simulink model "gm_hybrid_lht_vnl"  (R2019b)
settings: Solver=FixedStepDiscrete  StartTime=0.0  StopTime=inf  FixedStep=1/120e6  RelTol=1e-3
undefined symbols (not defined in the file or in its folder): bt, height, nTheta, width
libraries: hdlsllib x252, simulink x168, hdlmdlgenlib x11, dspsrcs4 x1
(part 10 of 12)

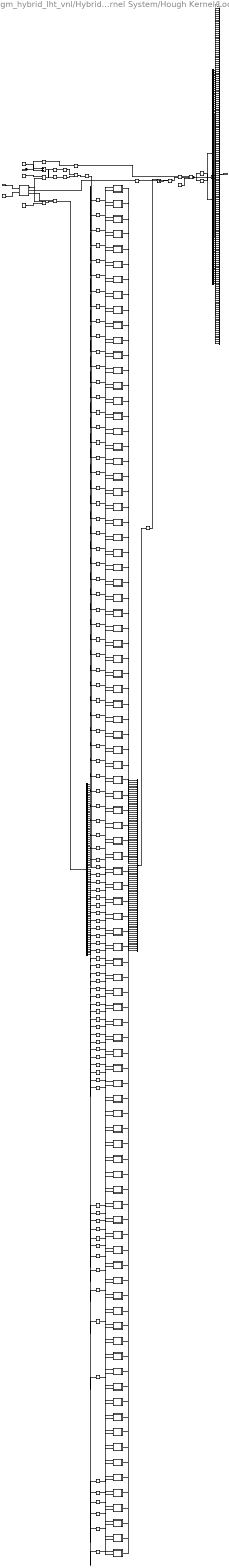
== system gm_hybrid_lht_vnl/Hybrid LHT/Hybrid LHT Kernel/Gradient Kernel System/Hough Kernel/Look Ahead Hough/Look Ahead Hough Symmetric ==
  Y : Inport  OutDataTypeStr=int8  PortDimensions=1  SampleTime=8.33333333333333e-09
  eol : Inport  Port=2  OutDataTypeStr=boolean  PortDimensions=1  SampleTime=8.33333333333333e-09
  AND1 : Logic  AllPortsSameDT=off  OutDataTypeStr=boolean  SampleTime=8.33333333333333e-09
  Add : Sum  AccumDataTypeStr=int8  OutDataTypeStr=int8  SampleTime=8.33333333333333e-09
  Compare To Constant : simulink/Logic and Bit Operations/Compare To Constant  relop===  const=fi(0,1,8,0,'hex','88')  OutDataTypeStr=boolean
  Constant : Constant  Value=90  OutDataTypeStr=uint8  SampleTime=-1
  Constant1 : Constant  OutDataTypeStr=int8  SampleTime=-1
  Delay_Switch : Switch  Criteria=u2 ~= 0  Threshold=double(0)  OutDataTypeStr=int8  SampleTime=8.33333333333333e-09
  HwModeRegister : Delay  DelayLength=double(1)  InitialCondition=0  SampleTime=8.33333333333333e-09
  HwModeRegister1 : Delay  DelayLength=double(1)  InitialCondition=0  SampleTime=8.33333333333333e-09
  MATLAB Function : Subsystem
  Multiport Switch : MultiPortSwitch  DataPortOrder=Zero-based contiguous  Inputs=2  DiagnosticForDefault=None  zeroidx=on  OutDataTypeStr=int8  SampleTime=8.33333333333333e-09
  PipelineRegister : Delay  DelayLength=double(1)  InitialCondition=0  SampleTime=8.33333333333333e-09
  Register Bank_instance1 : Subsystem
  Register Bank_instance10 : Subsystem
  Register Bank_instance11 : Subsystem
  Register Bank_instance12 : Subsystem
  Register Bank_instance13 : Subsystem
  Register Bank_instance14 : Subsystem
  Register Bank_instance15 : Subsystem
  Register Bank_instance16 : Subsystem
  Register Bank_instance17 : Subsystem
  Register Bank_instance18 : Subsystem
  Register Bank_instance19 : Subsystem
  Register Bank_instance2 : Subsystem
  Register Bank_instance20 : Subsystem
  Register Bank_instance21 : Subsystem
  Register Bank_instance22 : Subsystem
  Register Bank_instance23 : Subsystem
  Register Bank_instance24 : Subsystem
  Register Bank_instance25 : Subsystem
  Register Bank_instance26 : Subsystem
  Register Bank_instance27 : Subsystem
  Register Bank_instance28 : Subsystem
  Register Bank_instance29 : Subsystem
  Register Bank_instance3 : Subsystem
  Register Bank_instance30 : Subsystem
  Register Bank_instance31 : Subsystem
  Register Bank_instance32 : Subsystem
  Register Bank_instance33 : Subsystem
  Register Bank_instance34 : Subsystem
  Register Bank_instance35 : Subsystem
  Register Bank_instance36 : Subsystem
  Register Bank_instance37 : Subsystem
  Register Bank_instance38 : Subsystem
  Register Bank_instance39 : Subsystem
  Register Bank_instance4 : Subsystem
  Register Bank_instance40 : Subsystem
  Register Bank_instance41 : Subsystem
  Register Bank_instance42 : Subsystem
  Register Bank_instance43 : Subsystem
  Register Bank_instance44 : Subsystem
  Register Bank_instance45 : Subsystem
  Register Bank_instance46 : Subsystem
  Register Bank_instance47 : Subsystem
  Register Bank_instance48 : Subsystem
  Register Bank_instance49 : Subsystem
  Register Bank_instance5 : Subsystem
  Register Bank_instance50 : Subsystem
  Register Bank_instance51 : Subsystem
  Register Bank_instance52 : Subsystem
  Register Bank_instance53 : Subsystem
  Register Bank_instance54 : Subsystem
  Register Bank_instance55 : Subsystem
  Register Bank_instance56 : Subsystem
  Register Bank_instance57 : Subsystem
  Register Bank_instance58 : Subsystem
  Register Bank_instance59 : Subsystem
  Register Bank_instance6 : Subsystem
  Register Bank_instance60 : Subsystem
  Register Bank_instance61 : Subsystem
  Register Bank_instance62 : Subsystem
  Register Bank_instance63 : Subsystem
  Register Bank_instance64 : Subsystem
  Register Bank_instance65 : Subsystem
  Register Bank_instance66 : Subsystem
  Register Bank_instance67 : Subsystem
  Register Bank_instance68 : Subsystem
  Register Bank_instance69 : Subsystem
  Register Bank_instance7 : Subsystem
  Register Bank_instance70 : Subsystem
  Register Bank_instance71 : Subsystem
  Register Bank_instance72 : Subsystem
  Register Bank_instance73 : Subsystem
  Register Bank_instance74 : Subsystem
  Register Bank_instance75 : Subsystem
  Register Bank_instance76 : Subsystem
  Register Bank_instance77 : Subsystem
  Register Bank_instance78 : Subsystem
  Register Bank_instance79 : Subsystem
  Register Bank_instance8 : Subsystem
  Register Bank_instance80 : Subsystem
  Register Bank_instance81 : Subsystem
  Register Bank_instance82 : Subsystem
  Register Bank_instance83 : Subsystem
  Register Bank_instance84 : Subsystem
  Register Bank_instance85 : Subsystem
  Register Bank_instance86 : Subsystem
  Register Bank_instance87 : Subsystem
  Register Bank_instance88 : Subsystem
  Register Bank_instance89 : Subsystem
  Register Bank_instance9 : Subsystem
  Register Bank_instance90 : Subsystem
  Register Bank_instance91 : Subsystem
  Relational Operator : RelationalOperator  Operator===  OutDataTypeStr=boolean  SampleTime=8.33333333333333e-09  RndMeth=Nearest
  Selector : Selector  NumberOfDimensions=2  IndexMode=Zero-based  SampleTime=8.33333333333333e-09  IndexOptions=Index vector (dialog),Index vector (dialog)  Indices=double(0),double(90)  OutputSizes=double(1),double(1)
  Selector1 : Selector  NumberOfDimensions=2  IndexMode=Zero-based  SampleTime=8.33333333333333e-09  IndexOptions=Index vector (dialog),Index vector (port)  Indices=double(0),double(1)  OutputSizes=double(1),double(1)
  Selector2 : Selector  NumberOfDimensions=2  IndexMode=Zero-based  SampleTime=8.33333333333333e-09  IndexOptions=Index vector (dialog),Index vector (dialog)  Indices=double(0),double([0 1 2 3 4 5 6 7 8 9 10 11 12 13 14 15 16 17 18 19 20 21 22 23 24 25 26 27 28 29 30 31 32 33 34 35 36 37 38 39 40 41 42 43 44 45 46 47 48 49 50 51 52 53 54 55 56 57 58 59 60 61 62 63 64 65 66 67 68 69 70 71 72 73 74 75 76 77 78 79 80 81 82 83 84 85 86 87 88 89])  OutputSizes=double(1),double(1)
  Selector3 : Selector  NumberOfDimensions=2  IndexMode=Zero-based  SampleTime=8.33333333333333e-09  IndexOptions=Index vector (dialog),Index vector (dialog)  Indices=double(0),double([89 88 87 86 85 84 83 82 81 80 79 78 77 76 75 74 73 72 71 70 69 68 67 66 65 64 63 62 61 60 59 58 57 56 55 54 53 52 51 50 49 48 47 46 45 44 43 42 41 40 39 38 37 36 35 34 33 32 31 30 29 28 27 26 25 24 23 22 21 20 19 18 17 16 15 14 13 12 11 10 9 8 7 6 5 4 3 2 1])  OutputSizes=double(1),double(1)
  SineROM : Constant  Value=[0 0.0174560546875 0.034912109375 0.05230712890625 0.06976318359375 0.087158203125 0.10455322265625 0.12188720703125 0.13916015625 0.15643310546875 0.17364501953125 0.1907958984375 0.2078857421875 0.2249755859375 0.241943359375 0.2587890625 0.275634765625 0.2923583984375 0.30902099609375 0.3255615234375 0.342041015625 0.3583984375 0.3746337890625 0.3907470703125 0.40673828125 0.422607421875 0.4383544921875 0.4539794921875 0.469482421875 0.48480224609375 0.5 0.5150146484375 0.5299072265625 0.54461669921875 0.5592041015625 0.57354736328125 0.5877685546875 0.601806640625 0.61566162109375 0.62933349609375 0.64276123046875 0.65606689453125 0.66912841796875 0.6820068359375 0.69464111328125 0.70709228515625 0.7193603515625 0.7313232421875 0.7431640625 0.75469970703125 0.76605224609375 0.77716064453125 0.78802490234375 0.79864501953125 0.80902099609375 0.81915283203125 0.82904052734375 0.83868408203125 0.8480224609375 0.857177734375 0.86602783203125 0.8746337890625 0.8829345703125 0.8909912109375 0.8988037109375 0.90631103515625 0.91357421875 0.9205322265625 0.92718505859375 0.93359375 0.939697265625 0.94549560546875 0.9510498046875 0.956298828125 0.96124267578125 0.9659423828125 0.97027587890625 0.974365234375 0.9781494140625 0.98162841796875 0.98480224609375 0.9876708984375 0.99029541015625 0.9925537109375 0.9945068359375 0.9962158203125 0.99755859375 0.9986572265625 0.9993896484375 0.9998779296875 1]  VectorParams1D=off  OutDataTypeStr=fixdt(1, 16, 14)  SampleTime=-1
  Unit Delay Enabled Synchronous_lowered : Delay  DelayLength=double(1)  InitialCondition=0  SampleTime=8.33333333333333e-09
  Unit Delay Enabled Synchronous_out1 : hdlmdlgenlib/Buffer
      settings: SourceProductName=Simulink  SourceProductBaseCode=SL
  concatenate : Concatenate  NumInputs=180  Mode=Multidimensional array  ConcatenateDimension=2
  delayMatch{,1..92} (93 alike) : Delay  DelayLength=double(2)  InitialCondition=0  SampleTime=8.33333333333333e-09
  multiply : Product  Inputs=**  OutDataTypeStr=fixdt(1, 24, 14)  SampleTime=8.33333333333333e-09
  multiply_in0_buff : hdlmdlgenlib/Buffer
      settings: SourceProductName=Simulink  SourceProductBaseCode=SL
  multiply_in1_buff : hdlmdlgenlib/Buffer
      settings: SourceProductName=Simulink  SourceProductBaseCode=SL
  multiply_out_dtc : DataTypeConversion  OutDataTypeStr=int8  RndMeth=Round  SampleTime=8.33333333333333e-09
  row_0 : Constant  Value=[0 -2 -4 -6 -8 -10 -13 -15 -17 -19 -21 -23 -25 -27 -29 -31 -33 -35 -37 -39 -41 -43 -45 -47 -49 -51 -53 -54 -56 -58 -60 -62 -64 -65 -67 -69 -71 -72 -74 -76 -77 -79 -80 -82 -83 -85 -86 -88 -89 -91 -92 -93 -95 -96 -97 -98 -99 -101 -102 -103 -104 -105 -106 -107 -108 -109 -110 -110 -111 -112 -113 -113 -114 -115 -115 -116 -116 -117 -117 -118 -118 -119 -119 -119 -119 -120 -120 -120 -120 -120 -120]  VectorParams1D=off  OutDataTypeStr=int8  SampleTime=-1
  t : Demux  Outputs=89
  t1 : Demux  Outputs=90
  t2 : Concatenate  NumInputs=91
  t3 : Reshape  OutputDimensionality=Row vector (2-D)
  t4 : Demux  Outputs=91
  theta_index : Constant  Value=[0 1 2 3 4 5 6 7 8 9 10 11 12 13 14 15 16 17 18 19 20 21 22 23 24 25 26 27 28 29 30 31 32 33 34 35 36 37 38 39 40 41 42 43 44 45 46 47 48 49 50 51 52 53 54 55 56 57 58 59 60 61 62 63 64 65 66 67 68 69 70 71 72 73 74 75 76 77 78 79 80 81 82 83 84 85 86 87 88 89 90]  VectorParams1D=off  OutDataTypeStr=uint8  SampleTime=-1
  ysin : Outport  VectorParamsAs1DForOutWhenUnconnected=off
  wires:
  multiply_in1_buff/1 -> HwModeRegister1/1
  multiply_in0_buff/1 -> HwModeRegister/1
  HwModeRegister1/1 -> multiply/2
  HwModeRegister/1 -> multiply/1
  multiply/1 -> PipelineRegister/1
  t2/1 -> t3/1
  t1/90 -> concatenate/90
  t1/89 -> concatenate/89
  t1/88 -> concatenate/88
  t1/87 -> concatenate/87
  t1/86 -> concatenate/86
  t1/85 -> concatenate/85
  t1/84 -> concatenate/84
  t1/83 -> concatenate/83
  t1/82 -> concatenate/82
  t1/81 -> concatenate/81
  t1/80 -> concatenate/80
  t1/79 -> concatenate/79
  t1/78 -> concatenate/78
  t1/77 -> concatenate/77
  t1/76 -> concatenate/76
  t1/75 -> concatenate/75
  t1/74 -> concatenate/74
  t1/73 -> concatenate/73
  t1/72 -> concatenate/72
  t1/71 -> concatenate/71
  t1/70 -> concatenate/70
  t1/69 -> concatenate/69
  t1/68 -> concatenate/68
  t1/67 -> concatenate/67
  t1/66 -> concatenate/66
  t1/65 -> concatenate/65
  t1/64 -> concatenate/64
  t1/63 -> concatenate/63
  t1/62 -> concatenate/62
  t1/61 -> concatenate/61
  t1/60 -> concatenate/60
  t1/59 -> concatenate/59
  t1/58 -> concatenate/58
  t1/57 -> concatenate/57
  t1/56 -> concatenate/56
  t1/55 -> concatenate/55
  t1/54 -> concatenate/54
  t1/53 -> concatenate/53
  t1/52 -> concatenate/52
  t1/51 -> concatenate/51
  t1/50 -> concatenate/50
  t1/49 -> concatenate/49
  t1/48 -> concatenate/48
  t1/47 -> concatenate/47
  t1/46 -> concatenate/46
  t1/45 -> concatenate/45
  t1/44 -> concatenate/44
  t1/43 -> concatenate/43
  t1/42 -> concatenate/42
  t1/41 -> concatenate/41
  t1/40 -> concatenate/40
  t1/39 -> concatenate/39
  t1/38 -> concatenate/38
  t1/37 -> concatenate/37
  t1/36 -> concatenate/36
  t1/35 -> concatenate/35
  t1/34 -> concatenate/34
  t1/33 -> concatenate/33
  t1/32 -> concatenate/32
  t1/31 -> concatenate/31
  t1/30 -> concatenate/30
  t1/29 -> concatenate/29
  t1/28 -> concatenate/28
  t1/27 -> concatenate/27
  t1/26 -> concatenate/26
  t1/25 -> concatenate/25
  t1/24 -> concatenate/24
  t1/23 -> concatenate/23
  t1/22 -> concatenate/22
  t1/21 -> concatenate/21
  t1/20 -> concatenate/20
  t1/19 -> concatenate/19
  t1/18 -> concatenate/18
  t1/17 -> concatenate/17
  t1/16 -> concatenate/16
  t1/15 -> concatenate/15
  t1/14 -> concatenate/14
  t1/13 -> concatenate/13
  t1/12 -> concatenate/12
  t1/11 -> concatenate/11
  t1/10 -> concatenate/10
  t1/9 -> concatenate/9
  t1/8 -> concatenate/8
  t1/7 -> concatenate/7
  t1/6 -> concatenate/6
  t1/5 -> concatenate/5
  t1/4 -> concatenate/4
  t1/3 -> concatenate/3
  t1/2 -> concatenate/2
  t1/1 -> concatenate/1
  t/89 -> concatenate/180
  t/88 -> concatenate/179
  t/87 -> concatenate/178
  t/86 -> concatenate/177
  t/85 -> concatenate/176
  t/84 -> concatenate/175
  t/83 -> concatenate/174
  t/82 -> concatenate/173
  t/81 -> concatenate/172
  t/80 -> concatenate/171
  t/79 -> concatenate/170
  t/78 -> concatenate/169
  t/77 -> concatenate/168
  t/76 -> concatenate/167
  t/75 -> concatenate/166
  t/74 -> concatenate/165
  t/73 -> concatenate/164
  t/72 -> concatenate/163
  t/71 -> concatenate/162
  t/70 -> concatenate/161
  t/69 -> concatenate/160
  t/68 -> concatenate/159
  t/67 -> concatenate/158
  t/66 -> concatenate/157
  t/65 -> concatenate/156
  t/64 -> concatenate/155
  t/63 -> concatenate/154
  t/62 -> concatenate/153
  t/61 -> concatenate/152
  t/60 -> concatenate/151
  t/59 -> concatenate/150
  t/58 -> concatenate/149
  t/57 -> concatenate/148
  t/56 -> concatenate/147
  t/55 -> concatenate/146
  t/54 -> concatenate/145
  t/53 -> concatenate/144
  t/52 -> concatenate/143
  t/51 -> concatenate/142
  t/50 -> concatenate/141
  t/49 -> concatenate/140
  t/48 -> concatenate/139
  t/47 -> concatenate/138
  t/46 -> concatenate/137
  t/45 -> concatenate/136
  t/44 -> concatenate/135
  t/43 -> concatenate/134
  t/42 -> concatenate/133
  t/41 -> concatenate/132
  t/40 -> concatenate/131
  t/39 -> concatenate/130
  t/38 -> concatenate/129
  t/37 -> concatenate/128
  t/36 -> concatenate/127
  t/35 -> concatenate/126
  t/34 -> concatenate/125
  t/33 -> concatenate/124
  t/32 -> concatenate/123
  t/31 -> concatenate/122
  t/30 -> concatenate/121
  t/29 -> concatenate/120
  t/28 -> concatenate/119
  t/27 -> concatenate/118
  t/26 -> concatenate/117
  t/25 -> concatenate/116
  t/24 -> concatenate/115
  t/23 -> concatenate/114
  t/22 -> concatenate/113
  t/21 -> concatenate/112
  t/20 -> concatenate/111
  t/19 -> concatenate/110
  t/18 -> concatenate/109
  t/17 -> concatenate/108
  t/16 -> concatenate/107
  t/15 -> concatenate/106
  t/14 -> concatenate/105
  t/13 -> concatenate/104
  t/12 -> concatenate/103
  t/11 -> concatenate/102
  t/10 -> concatenate/101
  t/9 -> concatenate/100
  t/8 -> concatenate/99
  t/7 -> concatenate/98
  t/6 -> concatenate/97
  t/5 -> concatenate/96
  t/4 -> concatenate/95
  t/3 -> concatenate/94
  t/2 -> concatenate/93
  t/1 -> concatenate/92
  Register Bank_instance1/1(Data Out) -> t2/1
  Register Bank_instance2/1(Data Out) -> t2/2
  multiply_out_dtc/1 -> Register Bank_instance1/1(Data In), Register Bank_instance2/1(Data In), Register Bank_instance3/1(Data In), Register Bank_instance4/1(Data In), Register Bank_instance5/1(Data In), Register Bank_instance6/1(Data In), Register Bank_instance7/1(Data In), Register Bank_instance8/1(Data In), Register Bank_instance9/1(Data In), Register Bank_instance10/1(Data In), Register Bank_instance11/1(Data In), Register Bank_instance12/1(Data In), Register Bank_instance13/1(Data In), Register Bank_instance14/1(Data In), Register Bank_instance15/1(Data In), Register Bank_instance16/1(Data In), Register Bank_instance17/1(Data In), Register Bank_instance18/1(Data In), Register Bank_instance19/1(Data In), Register Bank_instance20/1(Data In), Register Bank_instance21/1(Data In), Register Bank_instance22/1(Data In), Register Bank_instance23/1(Data In), Register Bank_instance24/1(Data In), Register Bank_instance25/1(Data In), Register Bank_instance26/1(Data In), Register Bank_instance27/1(Data In), Register Bank_instance28/1(Data In), Register Bank_instance29/1(Data In), Register Bank_instance30/1(Data In), Register Bank_instance31/1(Data In), Register Bank_instance32/1(Data In), Register Bank_instance33/1(Data In), Register Bank_instance34/1(Data In), Register Bank_instance35/1(Data In), Register Bank_instance36/1(Data In), Register Bank_instance37/1(Data In), Register Bank_instance38/1(Data In), Register Bank_instance39/1(Data In), Register Bank_instance40/1(Data In), Register Bank_instance41/1(Data In), Register Bank_instance42/1(Data In), Register Bank_instance43/1(Data In), Register Bank_instance44/1(Data In), Register Bank_instance45/1(Data In), Register Bank_instance46/1(Data In), Register Bank_instance47/1(Data In), Register Bank_instance48/1(Data In), Register Bank_instance49/1(Data In), Register Bank_instance50/1(Data In), Register Bank_instance51/1(Data In), Register Bank_instance52/1(Data In), Register Bank_instance53/1(Data In), Register Bank_instance54/1(Data In), Register Bank_instance55/1(Data In), Register Bank_instance56/1(Data In), Register Bank_instance57/1(Data In), Register Bank_instance58/1(Data In), Register Bank_instance59/1(Data In), Register Bank_instance60/1(Data In), Register Bank_instance61/1(Data In), Register Bank_instance62/1(Data In), Register Bank_instance63/1(Data In), Register Bank_instance64/1(Data In), Register Bank_instance65/1(Data In), Register Bank_instance66/1(Data In), Register Bank_instance67/1(Data In), Register Bank_instance68/1(Data In), Register Bank_instance69/1(Data In), Register Bank_instance70/1(Data In), Register Bank_instance71/1(Data In), Register Bank_instance72/1(Data In), Register Bank_instance73/1(Data In), Register Bank_instance74/1(Data In), Register Bank_instance75/1(Data In), Register Bank_instance76/1(Data In), Register Bank_instance77/1(Data In), Register Bank_instance78/1(Data In), Register Bank_instance79/1(Data In), Register Bank_instance80/1(Data In), Register Bank_instance81/1(Data In), Register Bank_instance82/1(Data In), Register Bank_instance83/1(Data In), Register Bank_instance84/1(Data In), Register Bank_instance85/1(Data In), Register Bank_instance86/1(Data In), Register Bank_instance87/1(Data In), Register Bank_instance88/1(Data In), Register Bank_instance89/1(Data In), Register Bank_instance90/1(Data In), Register Bank_instance91/1(Data In)
  PipelineRegister/1 -> multiply_out_dtc/1
  Add/1 -> multiply_in1_buff/1
  Selector1/1 -> multiply_in0_buff/1
  Register Bank_instance91/1(Data Out) -> t2/91
  delayMatch92/1 -> Register Bank_instance91/2(Write Enable)
  t4/91 -> delayMatch92/1
  t4/90 -> delayMatch91/1
  t4/89 -> delayMatch90/1
  t4/88 -> delayMatch89/1
  t4/87 -> delayMatch88/1
  t4/86 -> delayMatch87/1
  t4/85 -> delayMatch86/1
  t4/84 -> delayMatch85/1
  t4/83 -> delayMatch84/1
  t4/82 -> delayMatch83/1
  t4/81 -> delayMatch82/1
  t4/80 -> delayMatch81/1
  t4/79 -> delayMatch80/1
  t4/78 -> delayMatch79/1
  t4/77 -> delayMatch78/1
  t4/76 -> delayMatch77/1
  t4/75 -> delayMatch76/1
  t4/74 -> delayMatch75/1
  t4/73 -> delayMatch74/1
  t4/72 -> delayMatch73/1
  t4/71 -> delayMatch72/1
  t4/70 -> delayMatch71/1
  t4/69 -> delayMatch70/1
  t4/68 -> delayMatch69/1
  t4/67 -> delayMatch68/1
  t4/66 -> delayMatch67/1
  t4/65 -> delayMatch66/1
  t4/64 -> delayMatch65/1
  t4/63 -> delayMatch64/1
  t4/62 -> delayMatch63/1
  t4/61 -> delayMatch62/1
  t4/60 -> delayMatch61/1
  t4/59 -> delayMatch60/1
  t4/58 -> delayMatch59/1
  t4/57 -> delayMatch58/1
  t4/56 -> delayMatch57/1
  t4/55 -> delayMatch56/1
  t4/54 -> delayMatch55/1
  t4/53 -> delayMatch54/1
  t4/52 -> delayMatch53/1
  t4/51 -> delayMatch52/1
  t4/50 -> delayMatch51/1
  t4/49 -> delayMatch50/1
  t4/48 -> delayMatch49/1
  t4/47 -> delayMatch48/1
  t4/46 -> delayMatch47/1
  t4/45 -> delayMatch46/1
  t4/44 -> delayMatch45/1
  t4/43 -> delayMatch44/1
  t4/42 -> delayMatch43/1
  t4/41 -> delayMatch42/1
  t4/40 -> delayMatch41/1
  t4/39 -> delayMatch40/1
  t4/38 -> delayMatch39/1
  t4/37 -> delayMatch38/1
  t4/36 -> delayMatch37/1
  t4/35 -> delayMatch36/1
  t4/34 -> delayMatch35/1
  t4/33 -> delayMatch34/1
  t4/32 -> delayMatch33/1
  t4/31 -> delayMatch32/1
  t4/30 -> delayMatch31/1
  t4/29 -> delayMatch30/1
  t4/28 -> delayMatch29/1
  t4/27 -> delayMatch28/1
  t4/26 -> delayMatch27/1
  t4/25 -> delayMatch26/1
  t4/24 -> delayMatch25/1
  t4/23 -> delayMatch24/1
  t4/22 -> delayMatch23/1
  t4/21 -> delayMatch22/1
  t4/20 -> delayMatch21/1
  t4/19 -> delayMatch20/1
  t4/18 -> delayMatch19/1
  t4/17 -> delayMatch18/1
  t4/16 -> delayMatch17/1
  t4/15 -> delayMatch16/1
  t4/14 -> delayMatch15/1
  t4/13 -> delayMatch14/1
  t4/12 -> delayMatch13/1
  t4/11 -> delayMatch12/1
  t4/10 -> delayMatch11/1
  t4/9 -> delayMatch10/1
  t4/8 -> delayMatch9/1
  t4/7 -> delayMatch8/1
  t4/6 -> delayMatch7/1
  t4/5 -> delayMatch6/1
  t4/4 -> delayMatch5/1
  t4/3 -> delayMatch4/1
  t4/2 -> delayMatch3/1
  t4/1 -> delayMatch2/1
  AND1/1 -> t4/1
  delayMatch91/1 -> Register Bank_instance90/2(Write Enable)
  Register Bank_instance90/1(Data Out) -> t2/90
  delayMatch90/1 -> Register Bank_instance89/2(Write Enable)
  Register Bank_instance89/1(Data Out) -> t2/89
  delayMatch89/1 -> Register Bank_instance88/2(Write Enable)
  Register Bank_instance88/1(Data Out) -> t2/88
  delayMatch88/1 -> Register Bank_instance87/2(Write Enable)
  Register Bank_instance87/1(Data Out) -> t2/87
  delayMatch87/1 -> Register Bank_instance86/2(Write Enable)
  Register Bank_instance86/1(Data Out) -> t2/86
  delayMatch86/1 -> Register Bank_instance85/2(Write Enable)
  Register Bank_instance85/1(Data Out) -> t2/85
  delayMatch85/1 -> Register Bank_instance84/2(Write Enable)
  Register Bank_instance84/1(Data Out) -> t2/84
  delayMatch84/1 -> Register Bank_instance83/2(Write Enable)
  Register Bank_instance83/1(Data Out) -> t2/83
  delayMatch83/1 -> Register Bank_instance82/2(Write Enable)
  Register Bank_instance82/1(Data Out) -> t2/82
  delayMatch82/1 -> Register Bank_instance81/2(Write Enable)
  Register Bank_instance81/1(Data Out) -> t2/81
  delayMatch81/1 -> Register Bank_instance80/2(Write Enable)
  Register Bank_instance80/1(Data Out) -> t2/80
  delayMatch80/1 -> Register Bank_instance79/2(Write Enable)
  Register Bank_instance79/1(Data Out) -> t2/79
  delayMatch79/1 -> Register Bank_instance78/2(Write Enable)
  Register Bank_instance78/1(Data Out) -> t2/78
  delayMatch78/1 -> Register Bank_instance77/2(Write Enable)
  Register Bank_instance77/1(Data Out) -> t2/77
  delayMatch77/1 -> Register Bank_instance76/2(Write Enable)
  Register Bank_instance76/1(Data Out) -> t2/76
  delayMatch76/1 -> Register Bank_instance75/2(Write Enable)
  Register Bank_instance75/1(Data Out) -> t2/75
  delayMatch75/1 -> Register Bank_instance74/2(Write Enable)
  Register Bank_instance74/1(Data Out) -> t2/74
  delayMatch74/1 -> Register Bank_instance73/2(Write Enable)
  Register Bank_instance73/1(Data Out) -> t2/73
  delayMatch73/1 -> Register Bank_instance72/2(Write Enable)
  Register Bank_instance72/1(Data Out) -> t2/72
  delayMatch72/1 -> Register Bank_instance71/2(Write Enable)
  Register Bank_instance71/1(Data Out) -> t2/71
  delayMatch71/1 -> Register Bank_instance70/2(Write Enable)
  Register Bank_instance70/1(Data Out) -> t2/70
  delayMatch70/1 -> Register Bank_instance69/2(Write Enable)
  Register Bank_instance69/1(Data Out) -> t2/69
  delayMatch69/1 -> Register Bank_instance68/2(Write Enable)
  Register Bank_instance68/1(Data Out) -> t2/68
  delayMatch68/1 -> Register Bank_instance67/2(Write Enable)
  Register Bank_instance67/1(Data Out) -> t2/67
  delayMatch67/1 -> Register Bank_instance66/2(Write Enable)
  Register Bank_instance66/1(Data Out) -> t2/66
  delayMatch66/1 -> Register Bank_instance65/2(Write Enable)
  Register Bank_instance65/1(Data Out) -> t2/65
  delayMatch65/1 -> Register Bank_instance64/2(Write Enable)
  Register Bank_instance64/1(Data Out) -> t2/64
  delayMatch64/1 -> Register Bank_instance63/2(Write Enable)
  Register Bank_instance63/1(Data Out) -> t2/63
  delayMatch63/1 -> Register Bank_instance62/2(Write Enable)
  Register Bank_instance62/1(Data Out) -> t2/62
  delayMatch62/1 -> Register Bank_instance61/2(Write Enable)
  Register Bank_instance61/1(Data Out) -> t2/61
  delayMatch61/1 -> Register Bank_instance60/2(Write Enable)
  Register Bank_instance60/1(Data Out) -> t2/60
  delayMatch60/1 -> Register Bank_instance59/2(Write Enable)
  Register Bank_instance59/1(Data Out) -> t2/59
  delayMatch59/1 -> Register Bank_instance58/2(Write Enable)
  Register Bank_instance58/1(Data Out) -> t2/58
  delayMatch58/1 -> Register Bank_instance57/2(Write Enable)
  Register Bank_instance57/1(Data Out) -> t2/57
  delayMatch57/1 -> Register Bank_instance56/2(Write Enable)
  Register Bank_instance56/1(Data Out) -> t2/56
  delayMatch56/1 -> Register Bank_instance55/2(Write Enable)
  Register Bank_instance55/1(Data Out) -> t2/55
  delayMatch55/1 -> Register Bank_instance54/2(Write Enable)
  Register Bank_instance54/1(Data Out) -> t2/54
  delayMatch54/1 -> Register Bank_instance53/2(Write Enable)
  Register Bank_instance53/1(Data Out) -> t2/53
  delayMatch53/1 -> Register Bank_instance52/2(Write Enable)
  Register Bank_instance52/1(Data Out) -> t2/52
  delayMatch52/1 -> Register Bank_instance51/2(Write Enable)
  Register Bank_instance51/1(Data Out) -> t2/51
  delayMatch51/1 -> Register Bank_instance50/2(Write Enable)
  Register Bank_instance50/1(Data Out) -> t2/50
  delayMatch50/1 -> Register Bank_instance49/2(Write Enable)
  Register Bank_instance49/1(Data Out) -> t2/49
  delayMatch49/1 -> Register Bank_instance48/2(Write Enable)
  Register Bank_instance48/1(Data Out) -> t2/48
  delayMatch48/1 -> Register Bank_instance47/2(Write Enable)
  Register Bank_instance47/1(Data Out) -> t2/47
  delayMatch47/1 -> Register Bank_instance46/2(Write Enable)
  Register Bank_instance46/1(Data Out) -> t2/46
  delayMatch46/1 -> Register Bank_instance45/2(Write Enable)
  Register Bank_instance45/1(Data Out) -> t2/45
  delayMatch45/1 -> Register Bank_instance44/2(Write Enable)
  Register Bank_instance44/1(Data Out) -> t2/44
  delayMatch44/1 -> Register Bank_instance43/2(Write Enable)
  Register Bank_instance43/1(Data Out) -> t2/43
  delayMatch43/1 -> Register Bank_instance42/2(Write Enable)
  Register Bank_instance42/1(Data Out) -> t2/42
  delayMatch42/1 -> Register Bank_instance41/2(Write Enable)
  Register Bank_instance41/1(Data Out) -> t2/41
  delayMatch41/1 -> Register Bank_instance40/2(Write Enable)
  Register Bank_instance40/1(Data Out) -> t2/40
  delayMatch40/1 -> Register Bank_instance39/2(Write Enable)
  Register Bank_instance39/1(Data Out) -> t2/39
  delayMatch39/1 -> Register Bank_instance38/2(Write Enable)
  Register Bank_instance38/1(Data Out) -> t2/38
  delayMatch38/1 -> Register Bank_instance37/2(Write Enable)
  Register Bank_instance37/1(Data Out) -> t2/37
  delayMatch37/1 -> Register Bank_instance36/2(Write Enable)
  Register Bank_instance36/1(Data Out) -> t2/36
  delayMatch36/1 -> Register Bank_instance35/2(Write Enable)
  Register Bank_instance35/1(Data Out) -> t2/35
  delayMatch35/1 -> Register Bank_instance34/2(Write Enable)
  Register Bank_instance34/1(Data Out) -> t2/34
  delayMatch34/1 -> Register Bank_instance33/2(Write Enable)
  Register Bank_instance33/1(Data Out) -> t2/33
  delayMatch33/1 -> Register Bank_instance32/2(Write Enable)
  Register Bank_instance32/1(Data Out) -> t2/32
  delayMatch32/1 -> Register Bank_instance31/2(Write Enable)
  Register Bank_instance31/1(Data Out) -> t2/31
  delayMatch31/1 -> Register Bank_instance30/2(Write Enable)
  Register Bank_instance30/1(Data Out) -> t2/30
  delayMatch30/1 -> Register Bank_instance29/2(Write Enable)
  Register Bank_instance29/1(Data Out) -> t2/29
  delayMatch29/1 -> Register Bank_instance28/2(Write Enable)
  Register Bank_instance28/1(Data Out) -> t2/28
  delayMatch28/1 -> Register Bank_instance27/2(Write Enable)
  Register Bank_instance27/1(Data Out) -> t2/27
  delayMatch27/1 -> Register Bank_instance26/2(Write Enable)
  Register Bank_instance26/1(Data Out) -> t2/26
  delayMatch26/1 -> Register Bank_instance25/2(Write Enable)
  Register Bank_instance25/1(Data Out) -> t2/25
  delayMatch25/1 -> Register Bank_instance24/2(Write Enable)
  Register Bank_instance24/1(Data Out) -> t2/24
  delayMatch24/1 -> Register Bank_instance23/2(Write Enable)
  Register Bank_instance23/1(Data Out) -> t2/23
  delayMatch23/1 -> Register Bank_instance22/2(Write Enable)
  Register Bank_instance22/1(Data Out) -> t2/22
  delayMatch22/1 -> Register Bank_instance21/2(Write Enable)
  Register Bank_instance21/1(Data Out) -> t2/21
  delayMatch21/1 -> Register Bank_instance20/2(Write Enable)
  Register Bank_instance20/1(Data Out) -> t2/20
  delayMatch20/1 -> Register Bank_instance19/2(Write Enable)
  Register Bank_instance19/1(Data Out) -> t2/19
  delayMatch19/1 -> Register Bank_instance18/2(Write Enable)
  Register Bank_instance18/1(Data Out) -> t2/18
  delayMatch18/1 -> Register Bank_instance17/2(Write Enable)
  Register Bank_instance17/1(Data Out) -> t2/17
  delayMatch17/1 -> Register Bank_instance16/2(Write Enable)
  Register Bank_instance16/1(Data Out) -> t2/16
  delayMatch16/1 -> Register Bank_instance15/2(Write Enable)
  Register Bank_instance15/1(Data Out) -> t2/15
  delayMatch15/1 -> Register Bank_instance14/2(Write Enable)
  Register Bank_instance14/1(Data Out) -> t2/14
  delayMatch14/1 -> Register Bank_instance13/2(Write Enable)
  Register Bank_instance13/1(Data Out) -> t2/13
  delayMatch13/1 -> Register Bank_instance12/2(Write Enable)
  Register Bank_instance12/1(Data Out) -> t2/12
  delayMatch12/1 -> Register Bank_instance11/2(Write Enable)
  Register Bank_instance11/1(Data Out) -> t2/11
  delayMatch11/1 -> Register Bank_instance10/2(Write Enable)
  Register Bank_instance10/1(Data Out) -> t2/10
  delayMatch10/1 -> Register Bank_instance9/2(Write Enable)
  Register Bank_instance9/1(Data Out) -> t2/9
  delayMatch9/1 -> Register Bank_instance8/2(Write Enable)
  Register Bank_instance8/1(Data Out) -> t2/8
  delayMatch8/1 -> Register Bank_instance7/2(Write Enable)
  Register Bank_instance7/1(Data Out) -> t2/7
  delayMatch7/1 -> Register Bank_instance6/2(Write Enable)
  Register Bank_instance6/1(Data Out) -> t2/6
  delayMatch6/1 -> Register Bank_instance5/2(Write Enable)
  Register Bank_instance5/1(Data Out) -> t2/5
  delayMatch5/1 -> Register Bank_instance4/2(Write Enable)
  Register Bank_instance4/1(Data Out) -> t2/4
  delayMatch4/1 -> Register Bank_instance3/2(Write Enable)
  Register Bank_instance3/1(Data Out) -> t2/3
  delayMatch3/1 -> Register Bank_instance2/2(Write Enable)
  delayMatch2/1 -> Register Bank_instance1/2(Write Enable)
  t3/1 -> Delay_Switch/1
  Delay_Switch/1 -> Unit Delay Enabled Synchronous_lowered/1
  delayMatch1/1 -> Delay_Switch/2
  Unit Delay Enabled Synchronous_lowered/1 -> Unit Delay Enabled Synchronous_out1/1, Delay_Switch/3
  Unit Delay Enabled Synchronous_out1/1 -> Multiport Switch/2
  Multiport Switch/1 -> Selector/1, Selector2/1, Selector3/1
  delayMatch/1 -> Multiport Switch/1
  Compare To Constant/1 -> delayMatch/1
  Selector3/1 -> t/1
  Selector/1 -> concatenate/91
  Selector2/1 -> t1/1
  MATLAB Function/2(sel) -> delayMatch1/1
  eol/1 -> MATLAB Function/1(eol)
  Y/1 -> Compare To Constant/1, Add/2
  theta_index/1 -> Relational Operator/2
  row_0/1 -> Multiport Switch/3
  SineROM/1 -> Selector1/1
  Relational Operator/1 -> AND1/2
  concatenate/1 -> ysin/1
  MATLAB Function/3(write) -> AND1/1
  MATLAB Function/1(index) -> Selector1/2, Relational Operator/1
  Constant1/1 -> Add/1
  Constant/1 -> MATLAB Function/2(ntheta)

== system gm_hybrid_lht_vnl/Hybrid LHT_vnl/Hybrid LHT Accumulator/Accumulator with Switches/Accumulator/Block RAM/Simple Dual Port RAM ==
  wr_data : Inport
  wr_addr : Inport  Port=2
  wr_en : Inport  Port=3
  rd_addr : Inport  Port=4
  Simple Dual Port RAM : hdlsllib/HDL RAMs/Simple Dual Port RAM  ram_size=ceil(log2(maxRho*2))
      settings: SourceProductName=Simulink  SourceProductBaseCode=SL
  rd_data : Outport
  wires:
  wr_data/1 -> Simple Dual Port RAM/1
  wr_addr/1 -> Simple Dual Port RAM/2
  wr_en/1 -> Simple Dual Port RAM/3
  rd_addr/1 -> Simple Dual Port RAM/4
  Simple Dual Port RAM/1 -> rd_data/1

== system gm_hybrid_lht_vnl/Hybrid LHT_vnl/Hybrid LHT Accumulator/Accumulator with Switches/Accumulator/Block RAM/Simple Dual Port RAM Generator ==
  wr_data : Inport
  wr_addr : Inport  Port=2
  wr_en : Inport  Port=3
  rd_addr : Inport  Port=4
  rd_address : hdlsllib/Logic and Bit Operations/Bit Slice  lidx=8  ridx=0
      settings: SourceProductName=Simulink  SourceProductBaseCode=SL
  simple_ram_0 : hdlsllib/HDL RAMs/Simple Dual Port RAM  ram_size=9
      settings: SourceProductName=Simulink  SourceProductBaseCode=SL
  wr_address : hdlsllib/Logic and Bit Operations/Bit Slice  lidx=8  ridx=0
      settings: SourceProductName=Simulink  SourceProductBaseCode=SL
  rd_data : Outport
  wires:
  simple_ram_0/1 -> rd_data/1
  rd_address/1 -> simple_ram_0/4
  rd_addr/1 -> rd_address/1
  wr_en/1 -> simple_ram_0/3
  wr_address/1 -> simple_ram_0/2
  wr_addr/1 -> wr_address/1
  wr_data/1 -> simple_ram_0/1

== system gm_hybrid_lht_vnl/Hybrid LHT_vnl/Hybrid LHT Kernel/Gradient Kernel System/Hough Kernel/Look Ahead Hough/Look Ahead Hough ==
  Y : Inport
  eol : Inport  Port=2
  AND1 : Logic  IconShape=distinctive  AllPortsSameDT=off  OutDataTypeStr=boolean
  Add : Sum  OutDataTypeStr=fixdt(1,ceil(log2(height)),0)
  Compare To Constant : simulink/Logic and Bit Operations/Compare To Constant  relop===  const=-height/2  OutDataTypeStr=boolean
  Constant : Constant  Value=nTheta-1  OutDataTypeStr=fixdt(0, ceil(log2(nTheta+1)), 0)  SampleTime=-1
  Constant1 : Constant  OutDataTypeStr=fixdt(1, ceil(log2(height)), 0);  SampleTime=-1
  MATLAB Function : MATLAB Function  TreatAsAtomicUnit=on
  Multiport Switch : MultiPortSwitch  DataPortOrder=Zero-based contiguous  Inputs=2  zeroidx=on
  Register Bank : Subsystem  TreatAsAtomicUnit=on
  Relational Operator : RelationalOperator  Operator===  OutDataTypeStr=boolean  RndMeth=Simplest
  Selector1 : Selector  NumberOfDimensions=2  IndexMode=Zero-based  InputPortWidth=3  IndexOptions=Index vector (dialog),Index vector (port)  Indices=0,1  OutputSizes=1,1
  SineROM : Constant  Value=fi(sin(deg2rad(theta)), 1, 16, 14)  VectorParams1D=off  OutDataTypeStr=fixdt(1,16,14)  SampleTime=-1
  Terminator : Terminator
  Unit Delay Enabled Synchronous : hdlsllib/Discrete/Unit Delay Enabled Synchronous  InitialCondition=0.0  SampleTime=-1
      settings: SourceProductName=Simulink  SourceProductBaseCode=SL
  multiply : Product  OutDataTypeStr=fixdt(1, ceil(log2(height)), 0);  RndMeth=Round
  row_0 : Constant  Value=round(-height/2*fi(sin(deg2rad(theta)), 1, 16, 14))  VectorParams1D=off  OutDataTypeStr=fixdt(1,ceil(log2(height)),0)  SampleTime=-1
  theta_index : Constant  Value=[0:1:nTheta-1]  VectorParams1D=off  OutDataTypeStr=fixdt(0,ceil(log2(max(theta)+1)),0)  SampleTime=-1
  ysin : Outport  VectorParamsAs1DForOutWhenUnconnected=off
  wires:
  row_0/1 -> Multiport Switch/3
  Add/1 -> multiply/2
  Y/1 -> Add/2, Compare To Constant/1
  Constant1/1 -> Add/1
  MATLAB Function/3(write) -> AND1/1
  Constant/1 -> MATLAB Function/2(ntheta)
  eol/1 -> MATLAB Function/1(eol)
  MATLAB Function/1(index) -> Selector1/2, Relational Operator/1
  Selector1/1 -> multiply/1
  multiply/1 -> Register Bank/1(Data In)
  theta_index/1 -> Relational Operator/2
  Relational Operator/1 -> AND1/2
  AND1/1 -> Register Bank/2(Write Enable)
  MATLAB Function/4(debug_state) -> Terminator/1
  Multiport Switch/1 -> ysin/1
  SineROM/1 -> Selector1/1
  MATLAB Function/2(sel) -> Unit Delay Enabled Synchronous/2
  Compare To Constant/1 -> Multiport Switch/1
  Register Bank/1(Data Out) -> Unit Delay Enabled Synchronous/1
  Unit Delay Enabled Synchronous/1 -> Multiport Switch/2

== system gm_hybrid_lht_vnl/Hybrid LHT_vnl/Hybrid LHT Kernel/Gradient Kernel System/Hough Kernel/Look Ahead Hough/Look Ahead Hough Symmetric ==
  Y : Inport
  eol : Inport  Port=2
  AND1 : Logic  IconShape=distinctive  AllPortsSameDT=off  OutDataTypeStr=boolean
  Add : Sum  OutDataTypeStr=fixdt(1,ceil(log2(height)),0)
  Compare To Constant : simulink/Logic and Bit Operations/Compare To Constant  relop===  const=-height/2  OutDataTypeStr=boolean
  Constant : Constant  Value=nTheta/2  OutDataTypeStr=fixdt(0, ceil(log2(nTheta+1)), 0)  SampleTime=-1
  Constant1 : Constant  OutDataTypeStr=fixdt(1, ceil(log2(height)), 0);  SampleTime=-1
  MATLAB Function : MATLAB Function  TreatAsAtomicUnit=on
  Matrix Concatenate : Concatenate  NumInputs=3  Mode=Multidimensional array  ConcatenateDimension=2
  Multiport Switch : MultiPortSwitch  DataPortOrder=Zero-based contiguous  Inputs=2  zeroidx=on
  Register Bank : Subsystem  TreatAsAtomicUnit=on
  Relational Operator : RelationalOperator  Operator===  OutDataTypeStr=boolean  RndMeth=Simplest
  Selector : Selector  NumberOfDimensions=2  IndexMode=Zero-based  InputPortWidth=3  IndexOptions=Index vector (dialog),Index vector (dialog)  Indices=0,nTheta/2  OutputSizes=1,1
  Selector1 : Selector  NumberOfDimensions=2  IndexMode=Zero-based  InputPortWidth=3  IndexOptions=Index vector (dialog),Index vector (port)  Indices=0,1  OutputSizes=1,1
  Selector2 : Selector  NumberOfDimensions=2  IndexMode=Zero-based  InputPortWidth=3  IndexOptions=Index vector (dialog),Index vector (dialog)  Indices=0,[0:1:nTheta/2-1]  OutputSizes=1,1
  Selector3 : Selector  NumberOfDimensions=2  IndexMode=Zero-based  InputPortWidth=3  IndexOptions=Index vector (dialog),Index vector (dialog)  Indices=0,[nTheta/2-1:-1:1]  OutputSizes=1,1
  SineROM : Constant  Value=fi(sin(deg2rad(bt.theta(1:1:bt.nTheta/2+1))), 1, 16, 14)  VectorParams1D=off  OutDataTypeStr=fixdt(1,16,14)  SampleTime=-1
  Terminator : Terminator
  Unit Delay Enabled Synchronous : hdlsllib/Discrete/Unit Delay Enabled Synchronous  InitialCondition=0.0  SampleTime=-1
      settings: SourceProductName=Simulink  SourceProductBaseCode=SL
  multiply : Product  OutDataTypeStr=fixdt(1, ceil(log2(height)), 0);  RndMeth=Round
  row_0 : Constant  Value=round(-height/2*fi(sin(deg2rad(theta(1:1:nTheta/2+1))), 1, 16, 14))  VectorParams1D=off  OutDataTypeStr=fixdt(1,ceil(log2(height)),0)  SampleTime=-1
  theta_index : Constant  Value=[0:1:nTheta/2]  VectorParams1D=off  OutDataTypeStr=fixdt(0,ceil(log2(max(theta)+1)),0)  SampleTime=-1
  ysin : Outport  VectorParamsAs1DForOutWhenUnconnected=off
  wires:
  Selector3/1 -> Matrix Concatenate/3
  Selector2/1 -> Matrix Concatenate/1
  Multiport Switch/1 -> Selector2/1, Selector/1, Selector3/1
  Selector/1 -> Matrix Concatenate/2
  Matrix Concatenate/1 -> ysin/1
  Unit Delay Enabled Synchronous/1 -> Multiport Switch/2
  Register Bank/1(Data Out) -> Unit Delay Enabled Synchronous/1
  Compare To Constant/1 -> Multiport Switch/1
  MATLAB Function/2(sel) -> Unit Delay Enabled Synchronous/2
  SineROM/1 -> Selector1/1
  MATLAB Function/4(debug_state) -> Terminator/1
  AND1/1 -> Register Bank/2(Write Enable)
  Relational Operator/1 -> AND1/2
  theta_index/1 -> Relational Operator/2
  multiply/1 -> Register Bank/1(Data In)
  Selector1/1 -> multiply/1
  MATLAB Function/1(index) -> Relational Operator/1, Selector1/2
  eol/1 -> MATLAB Function/1(eol)
  Constant/1 -> MATLAB Function/2(ntheta)
  MATLAB Function/3(write) -> AND1/1
  Constant1/1 -> Add/1
  Y/1 -> Compare To Constant/1, Add/2
  Add/1 -> multiply/2
  row_0/1 -> Multiport Switch/3

== system gm_hybrid_lht_vnl/Hybrid LHT/Hybrid LHT Kernel/Gradient Kernel System/Hough Kernel/Look Ahead Hough/Look Ahead Hough Symmetric/MATLAB Function ==
  eol : Inport  OutDataTypeStr=boolean  PortDimensions=1  SampleTime=8.33333333333333e-09
  ntheta : Inport  Port=2  OutDataTypeStr=uint8  PortDimensions=1  SampleTime=8.33333333333333e-09
  MATLAB Function : MATLAB Function  TreatAsAtomicUnit=on
  index : Outport  VectorParamsAs1DForOutWhenUnconnected=off
  sel : Outport  Port=2  VectorParamsAs1DForOutWhenUnconnected=off
  write : Outport  Port=3  VectorParamsAs1DForOutWhenUnconnected=off
  wires:
  ntheta/1 -> MATLAB Function/2(ntheta)
  eol/1 -> MATLAB Function/1(eol)
  MATLAB Function/3(write) -> write/1
  MATLAB Function/2(sel) -> sel/1
  MATLAB Function/1(index) -> index/1

== system gm_hybrid_lht_vnl/Hybrid LHT/Hybrid LHT Kernel/Gradient Kernel System/Hough Kernel/Look Ahead Hough/Look Ahead Hough Symmetric/Register Bank_instance1 ==
  Data In : Inport  OutDataTypeStr=int8  PortDimensions=1  SampleTime=8.33333333333333e-09
  Write Enable : Inport  Port=2  OutDataTypeStr=boolean  PortDimensions=1  SampleTime=8.33333333333333e-09
  Delay_Switch : Switch  Criteria=u2 ~= 0  Threshold=double(0)  OutDataTypeStr=int8  SampleTime=8.33333333333333e-09
  Unit Delay Enabled Synchronous_lowered : Delay  DelayLength=double(1)  InitialCondition=0  SampleTime=8.33333333333333e-09
  Data Out : Outport
  wires:
  Unit Delay Enabled Synchronous_lowered/1 -> Data Out/1, Delay_Switch/3
  Data In/1 -> Delay_Switch/1
  Write Enable/1 -> Delay_Switch/2
  Delay_Switch/1 -> Unit Delay Enabled Synchronous_lowered/1

== system gm_hybrid_lht_vnl/Hybrid LHT/Hybrid LHT Kernel/Gradient Kernel System/Hough Kernel/Look Ahead Hough/Look Ahead Hough Symmetric/Register Bank_instance10 ==
  Data In : Inport  OutDataTypeStr=int8  PortDimensions=1  SampleTime=8.33333333333333e-09
  Write Enable : Inport  Port=2  OutDataTypeStr=boolean  PortDimensions=1  SampleTime=8.33333333333333e-09
  Delay_Switch : Switch  Criteria=u2 ~= 0  Threshold=double(0)  OutDataTypeStr=int8  SampleTime=8.33333333333333e-09
  Unit Delay Enabled Synchronous_lowered : Delay  DelayLength=double(1)  InitialCondition=0  SampleTime=8.33333333333333e-09
  Data Out : Outport
  wires:
  Unit Delay Enabled Synchronous_lowered/1 -> Data Out/1, Delay_Switch/3
  Data In/1 -> Delay_Switch/1
  Write Enable/1 -> Delay_Switch/2
  Delay_Switch/1 -> Unit Delay Enabled Synchronous_lowered/1

== system gm_hybrid_lht_vnl/Hybrid LHT/Hybrid LHT Kernel/Gradient Kernel System/Hough Kernel/Look Ahead Hough/Look Ahead Hough Symmetric/Register Bank_instance11 ==
  Data In : Inport  OutDataTypeStr=int8  PortDimensions=1  SampleTime=8.33333333333333e-09
  Write Enable : Inport  Port=2  OutDataTypeStr=boolean  PortDimensions=1  SampleTime=8.33333333333333e-09
  Delay_Switch : Switch  Criteria=u2 ~= 0  Threshold=double(0)  OutDataTypeStr=int8  SampleTime=8.33333333333333e-09
  Unit Delay Enabled Synchronous_lowered : Delay  DelayLength=double(1)  InitialCondition=0  SampleTime=8.33333333333333e-09
  Data Out : Outport
  wires:
  Unit Delay Enabled Synchronous_lowered/1 -> Data Out/1, Delay_Switch/3
  Data In/1 -> Delay_Switch/1
  Write Enable/1 -> Delay_Switch/2
  Delay_Switch/1 -> Unit Delay Enabled Synchronous_lowered/1

== system gm_hybrid_lht_vnl/Hybrid LHT/Hybrid LHT Kernel/Gradient Kernel System/Hough Kernel/Look Ahead Hough/Look Ahead Hough Symmetric/Register Bank_instance12 ==
  Data In : Inport  OutDataTypeStr=int8  PortDimensions=1  SampleTime=8.33333333333333e-09
  Write Enable : Inport  Port=2  OutDataTypeStr=boolean  PortDimensions=1  SampleTime=8.33333333333333e-09
  Delay_Switch : Switch  Criteria=u2 ~= 0  Threshold=double(0)  OutDataTypeStr=int8  SampleTime=8.33333333333333e-09
  Unit Delay Enabled Synchronous_lowered : Delay  DelayLength=double(1)  InitialCondition=0  SampleTime=8.33333333333333e-09
  Data Out : Outport
  wires:
  Unit Delay Enabled Synchronous_lowered/1 -> Data Out/1, Delay_Switch/3
  Data In/1 -> Delay_Switch/1
  Write Enable/1 -> Delay_Switch/2
  Delay_Switch/1 -> Unit Delay Enabled Synchronous_lowered/1

== system gm_hybrid_lht_vnl/Hybrid LHT/Hybrid LHT Kernel/Gradient Kernel System/Hough Kernel/Look Ahead Hough/Look Ahead Hough Symmetric/Register Bank_instance13 ==
  Data In : Inport  OutDataTypeStr=int8  PortDimensions=1  SampleTime=8.33333333333333e-09
  Write Enable : Inport  Port=2  OutDataTypeStr=boolean  PortDimensions=1  SampleTime=8.33333333333333e-09
  Delay_Switch : Switch  Criteria=u2 ~= 0  Threshold=double(0)  OutDataTypeStr=int8  SampleTime=8.33333333333333e-09
  Unit Delay Enabled Synchronous_lowered : Delay  DelayLength=double(1)  InitialCondition=0  SampleTime=8.33333333333333e-09
  Data Out : Outport
  wires:
  Unit Delay Enabled Synchronous_lowered/1 -> Data Out/1, Delay_Switch/3
  Data In/1 -> Delay_Switch/1
  Write Enable/1 -> Delay_Switch/2
  Delay_Switch/1 -> Unit Delay Enabled Synchronous_lowered/1

== system gm_hybrid_lht_vnl/Hybrid LHT/Hybrid LHT Kernel/Gradient Kernel System/Hough Kernel/Look Ahead Hough/Look Ahead Hough Symmetric/Register Bank_instance14 ==
  Data In : Inport  OutDataTypeStr=int8  PortDimensions=1  SampleTime=8.33333333333333e-09
  Write Enable : Inport  Port=2  OutDataTypeStr=boolean  PortDimensions=1  SampleTime=8.33333333333333e-09
  Delay_Switch : Switch  Criteria=u2 ~= 0  Threshold=double(0)  OutDataTypeStr=int8  SampleTime=8.33333333333333e-09
  Unit Delay Enabled Synchronous_lowered : Delay  DelayLength=double(1)  InitialCondition=0  SampleTime=8.33333333333333e-09
  Data Out : Outport
  wires:
  Unit Delay Enabled Synchronous_lowered/1 -> Data Out/1, Delay_Switch/3
  Data In/1 -> Delay_Switch/1
  Write Enable/1 -> Delay_Switch/2
  Delay_Switch/1 -> Unit Delay Enabled Synchronous_lowered/1

== system gm_hybrid_lht_vnl/Hybrid LHT/Hybrid LHT Kernel/Gradient Kernel System/Hough Kernel/Look Ahead Hough/Look Ahead Hough Symmetric/Register Bank_instance15 ==
  Data In : Inport  OutDataTypeStr=int8  PortDimensions=1  SampleTime=8.33333333333333e-09
  Write Enable : Inport  Port=2  OutDataTypeStr=boolean  PortDimensions=1  SampleTime=8.33333333333333e-09
  Delay_Switch : Switch  Criteria=u2 ~= 0  Threshold=double(0)  OutDataTypeStr=int8  SampleTime=8.33333333333333e-09
  Unit Delay Enabled Synchronous_lowered : Delay  DelayLength=double(1)  InitialCondition=0  SampleTime=8.33333333333333e-09
  Data Out : Outport
  wires:
  Unit Delay Enabled Synchronous_lowered/1 -> Data Out/1, Delay_Switch/3
  Data In/1 -> Delay_Switch/1
  Write Enable/1 -> Delay_Switch/2
  Delay_Switch/1 -> Unit Delay Enabled Synchronous_lowered/1

== system gm_hybrid_lht_vnl/Hybrid LHT/Hybrid LHT Kernel/Gradient Kernel System/Hough Kernel/Look Ahead Hough/Look Ahead Hough Symmetric/Register Bank_instance16 ==
  Data In : Inport  OutDataTypeStr=int8  PortDimensions=1  SampleTime=8.33333333333333e-09
  Write Enable : Inport  Port=2  OutDataTypeStr=boolean  PortDimensions=1  SampleTime=8.33333333333333e-09
  Delay_Switch : Switch  Criteria=u2 ~= 0  Threshold=double(0)  OutDataTypeStr=int8  SampleTime=8.33333333333333e-09
  Unit Delay Enabled Synchronous_lowered : Delay  DelayLength=double(1)  InitialCondition=0  SampleTime=8.33333333333333e-09
  Data Out : Outport
  wires:
  Unit Delay Enabled Synchronous_lowered/1 -> Data Out/1, Delay_Switch/3
  Data In/1 -> Delay_Switch/1
  Write Enable/1 -> Delay_Switch/2
  Delay_Switch/1 -> Unit Delay Enabled Synchronous_lowered/1

== system gm_hybrid_lht_vnl/Hybrid LHT/Hybrid LHT Kernel/Gradient Kernel System/Hough Kernel/Look Ahead Hough/Look Ahead Hough Symmetric/Register Bank_instance17 ==
  Data In : Inport  OutDataTypeStr=int8  PortDimensions=1  SampleTime=8.33333333333333e-09
  Write Enable : Inport  Port=2  OutDataTypeStr=boolean  PortDimensions=1  SampleTime=8.33333333333333e-09
  Delay_Switch : Switch  Criteria=u2 ~= 0  Threshold=double(0)  OutDataTypeStr=int8  SampleTime=8.33333333333333e-09
  Unit Delay Enabled Synchronous_lowered : Delay  DelayLength=double(1)  InitialCondition=0  SampleTime=8.33333333333333e-09
  Data Out : Outport
  wires:
  Unit Delay Enabled Synchronous_lowered/1 -> Data Out/1, Delay_Switch/3
  Data In/1 -> Delay_Switch/1
  Write Enable/1 -> Delay_Switch/2
  Delay_Switch/1 -> Unit Delay Enabled Synchronous_lowered/1

== system gm_hybrid_lht_vnl/Hybrid LHT/Hybrid LHT Kernel/Gradient Kernel System/Hough Kernel/Look Ahead Hough/Look Ahead Hough Symmetric/Register Bank_instance18 ==
  Data In : Inport  OutDataTypeStr=int8  PortDimensions=1  SampleTime=8.33333333333333e-09
  Write Enable : Inport  Port=2  OutDataTypeStr=boolean  PortDimensions=1  SampleTime=8.33333333333333e-09
  Delay_Switch : Switch  Criteria=u2 ~= 0  Threshold=double(0)  OutDataTypeStr=int8  SampleTime=8.33333333333333e-09
  Unit Delay Enabled Synchronous_lowered : Delay  DelayLength=double(1)  InitialCondition=0  SampleTime=8.33333333333333e-09
  Data Out : Outport
  wires:
  Unit Delay Enabled Synchronous_lowered/1 -> Data Out/1, Delay_Switch/3
  Data In/1 -> Delay_Switch/1
  Write Enable/1 -> Delay_Switch/2
  Delay_Switch/1 -> Unit Delay Enabled Synchronous_lowered/1

== system gm_hybrid_lht_vnl/Hybrid LHT/Hybrid LHT Kernel/Gradient Kernel System/Hough Kernel/Look Ahead Hough/Look Ahead Hough Symmetric/Register Bank_instance19 ==
  Data In : Inport  OutDataTypeStr=int8  PortDimensions=1  SampleTime=8.33333333333333e-09
  Write Enable : Inport  Port=2  OutDataTypeStr=boolean  PortDimensions=1  SampleTime=8.33333333333333e-09
  Delay_Switch : Switch  Criteria=u2 ~= 0  Threshold=double(0)  OutDataTypeStr=int8  SampleTime=8.33333333333333e-09
  Unit Delay Enabled Synchronous_lowered : Delay  DelayLength=double(1)  InitialCondition=0  SampleTime=8.33333333333333e-09
  Data Out : Outport
  wires:
  Unit Delay Enabled Synchronous_lowered/1 -> Data Out/1, Delay_Switch/3
  Data In/1 -> Delay_Switch/1
  Write Enable/1 -> Delay_Switch/2
  Delay_Switch/1 -> Unit Delay Enabled Synchronous_lowered/1
